simulink model "internalprop"  (R2023a)
settings: Solver=VariableStepAuto  StartTime=0.0  StopTime=tfin  RelTol=1e-3
values from neighbouring files (symbols this model uses):
  diam = [8,6,1/8]    [internalpropcode.m]
  g = 9.81    [internalpropcode.m]
  gama = 1.4    [internalpropcode.m]
  m = 15    [internalpropcode.m]
  v0 = 175    [internalpropcode.m]
  z0 = 0    [internalpropcode.m]
settings Model: Creator=Niko  LastModifiedBy=Niko
settings DataIOCC: SaveFormat=Array  SaveOutput=off  SignalLogging=off  DSMLogging=off  SaveTime=off  ReturnWorkspaceOutputs=off

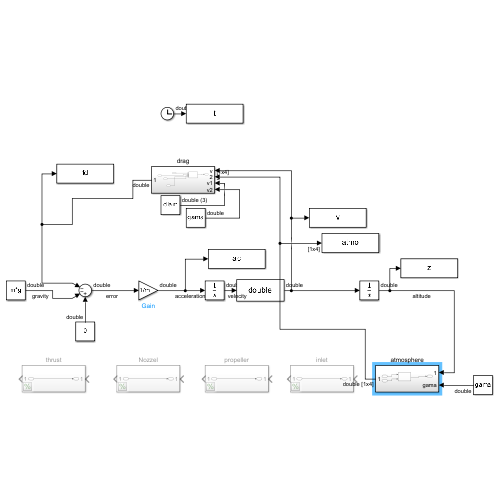
[thumbnail: Simulink's stored preview of the top-level diagram]
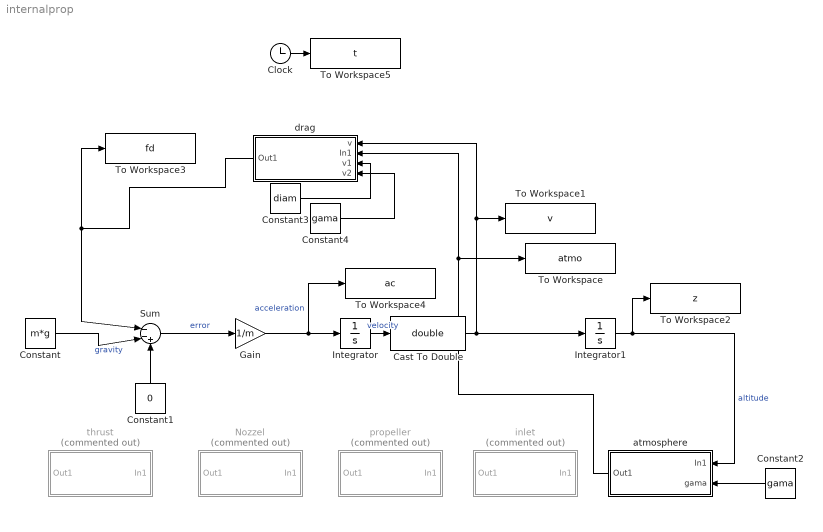
== system internalprop ==
  Cast To Double : DataTypeConversion  OutDataTypeStr=double  SaturateOnIntegerOverflow=off  RndMeth=Floor
  Clock : Clock
  Constant : Constant  Value=m*g
  Constant1 : Constant  Value=0
  Constant2 : Constant  Value=gama
  Constant3 : Constant  Value=diam
  Constant4 : Constant  Value=gama
  Gain : Gain  Gain=1/m
  Integrator : Integrator  InitialCondition=v0
  Integrator1 : Integrator  InitialCondition=z0
  Nozzel : Subsystem  Commented=on
  Sum : Sum  Inputs=|--+
  To Workspace : ToWorkspace  VariableName=atmo  SampleTime=-1
      settings: Save2DSignal=2-D array (concatenate along first dimension)
  To Workspace1 : ToWorkspace  VariableName=v  SampleTime=-1
      settings: Save2DSignal=2-D array (concatenate along first dimension)
  To Workspace2 : ToWorkspace  VariableName=z  SampleTime=-1
      settings: Save2DSignal=2-D array (concatenate along first dimension)
  To Workspace3 : ToWorkspace  VariableName=fd  SampleTime=-1
      settings: Save2DSignal=2-D array (concatenate along first dimension)
  To Workspace4 : ToWorkspace  VariableName=ac  SampleTime=-1
      settings: Save2DSignal=2-D array (concatenate along first dimension)
  To Workspace5 : ToWorkspace  VariableName=t  SampleTime=-1
      settings: Save2DSignal=2-D array (concatenate along first dimension)
  atmosphere : Subsystem
  drag : Subsystem
  inlet : Subsystem  Commented=on
  propeller : Subsystem  Commented=on
  thrust : Subsystem  Commented=on
  wires:
  Integrator/1 -> Cast To Double/1  "velocity"
  Integrator1/1 -> To Workspace2/1, atmosphere/1(In1)  "altitude"
  Gain/1 -> To Workspace4/1, Integrator/1  "acceleration"
  Sum/1 -> Gain/1  "error"
  Constant/1 -> Sum/2  "gravity"
  atmosphere/1(Out1) -> To Workspace/1, drag/2(In1)
  Constant1/1 -> Sum/3
  Clock/1 -> To Workspace5/1
  Constant2/1 -> atmosphere/2(gama)
  Cast To Double/1 -> drag/1(v), To Workspace1/1, Integrator1/1
  Constant3/1 -> drag/3(v1)
  Constant4/1 -> drag/4(v2)
  drag/1(Out1) -> To Workspace3/1, Sum/1

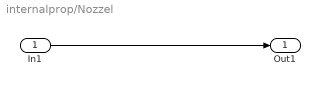
== system internalprop/Nozzel ==
  In1 : Inport
  Out1 : Outport
  wires:
  In1/1 -> Out1/1

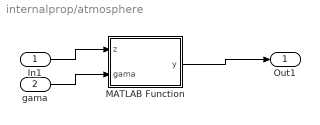
== system internalprop/atmosphere ==
  In1 : Inport
  gama : Inport  Port=2
  MATLAB Function : MATLAB Function  TreatAsAtomicUnit=on
  Out1 : Outport
  wires:
  In1/1 -> MATLAB Function/1(z)
  MATLAB Function/1(y) -> Out1/1
  gama/1 -> MATLAB Function/2(gama)

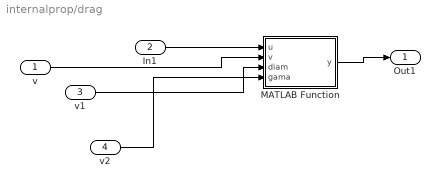
== system internalprop/drag ==
  v : Inport
  In1 : Inport  Port=2
  v1 : Inport  Port=3
  v2 : Inport  Port=4
  MATLAB Function : MATLAB Function  TreatAsAtomicUnit=on
  Out1 : Outport
  wires:
  In1/1 -> MATLAB Function/1(u)
  MATLAB Function/1(y) -> Out1/1
  v/1 -> MATLAB Function/2(v)
  v1/1 -> MATLAB Function/3(diam)
  v2/1 -> MATLAB Function/4(gama)

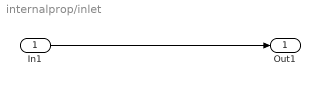
== system internalprop/inlet ==
  In1 : Inport
  Out1 : Outport
  wires:
  In1/1 -> Out1/1

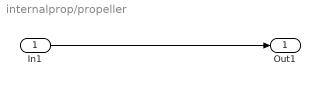
== system internalprop/propeller ==
  In1 : Inport
  Out1 : Outport
  wires:
  In1/1 -> Out1/1

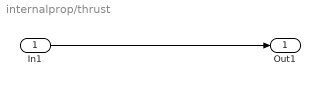
== system internalprop/thrust ==
  In1 : Inport
  Out1 : Outport
  wires:
  In1/1 -> Out1/1

== matlab function internalprop/drag/MATLAB Function ==
  data: u input; y output; v input; diam input; gama input
function y = fcn(u,v,diam,gama)
i=1;
y=0;
mach=double(v/u(3));
cdrr=cdr();
for j=1:1:size(cdrr,1)
	if mach >= cdrr(j,1) && mach < cdrr(j+1,1)
		i = j;
   % elseif mach>cdrr(0,end) || mach<cdrr(0,0)
    %    break;
    end
end
r= (cdrr(i,1) -mach)/(cdrr(i,1) - cdrr(i+1,1));
cd= cdrr(i+1,2)*r +cdrr(i,2)*(1-r);
y = double((double(diam(1)*diam(1))*pi* cd*(.5*u(4)/((1/(1+.5*(gama-1)*mach*mach)))^(1/(gama-1)))*double(v*v))/4);
end

== matlab function internalprop/atmosphere/MATLAB Function ==
  data: z input; y output; gama input
function y = fcn(z,gama)
%gama=1.4;
% y=zeros(4);
%[T,a,p,rho,nu] = atmosisa(z, extended=true);
z=z/0.3048;
T = 518.6;
	if z <= 36152. % #          // Troposphere
		T = 518.6 - 3.56 * z/1000. ;
    elseif z >= 36152. && z <= 82345.  %#  // Stratosphere
		T = 389.98 ;
    elseif z >= 82345. && z <= 155348.           
		T = 389.98 + 1.645 * (z-82345.)/1000. ;
    elseif z >= 155348. && z <= 175346.           
		T = 508.788 ;
    elseif z >= 175346. && z <= 262448.          
		T = 508.788 - 2.46888 * (z-175346.)/1000. ;
    elseif z>262448.
		T=0;
    end
rgas = 1718.;
a=((gama*rgas*T)^.5)*0.3048;
T=T*5/9;
z=z*0.3048/1000; %#altitude in km
%	#altitudes (km):
	h = [ 0, 25, 30, 40, 50, 60, 70, 80, 90, 100, 110, 120, 130, 140, 150, 180, 200, 250, 300, 350, 400, 450, 500, 600, 700, 800, 900, 1000];
%	#Corresponding densities (kg/m^3) from USSA76:
	r = [1.225, 4.008e-2, 1.841e-2, 3.996e-3, 1.027e-3, 3.097e-4, 8.283e-5, 1.846e-5, 3.416e-6, 5.606e-7, 9.708e-8, 2.222e-8, 8.152e-9, 3.831e-9, 2.076e-9, 5.194e-10, 2.541e-10, 6.073e-11, 1.916e-11, 7.014e-12, 2.803e-12, 1.184e-12, 5.215e-13, 1.137e-13, 3.070e-14, 1.136e-14, 5.759e-15, 3.561e-15];
%	#Scale heights (km):
	H = [ 7.310, 6.427, 6.546, 7.360, 8.342, 7.583, 6.661, 5.927, 5.533, 5.703, 6.782, 9.973, 13.243, 16.322, 21.652, 27.974, 34.934, 43.342, 49.755, 54.513, 58.019, 60.980, 65.654, 76.377, 100.587, 147.203, 208.020];
%	#Handle altitudes outside of the range:
	if z > 1000
	    z = 1000;
    elseif z < 0
	    z = 0;
    end
	%#Determine the interpolation interval:
	i=0;
	for j =1:28
        if z >= h(j) && z < h(j+1)
	        i = j;
        end
    end
	if z == 1000
	    i = 28;
    end
%	#Exponential interpolation:
	rho = r(i)*exp(-(z - h(i))/H(i));
R = 286.;
p=R*T*rho;
y=[T,p,a,rho];
